simulink library "calcTetherEndNodesStates"  (R2018b)
settings: Solver=VariableStepAuto  StartTime=0.0  StopTime=10.0  RelTol=1e-3
undefined symbols (not defined in the file): attchPtMat, class_thr, numTethers
libraries: vrlib x1, eulAng2RotMat_ul x1
settings Model: Creator=Ayaz  LastModifiedBy=Ayaz

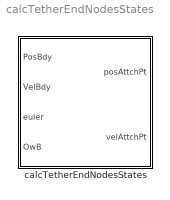
== system calcTetherEndNodesStates ==
  calcTetherEndNodesStates : Subsystem  TreatAsAtomicUnit=on  mask{thr_struct=class_thr, attach_point=Ground station}
      mask prompts: thr_struct "Tether class variable name"; attach_point "Choose attachment point"
      mask init:
      | sumTetherForcesAndMoments_init
      mask TypeOptions attach_point: Ground station | Lifting body

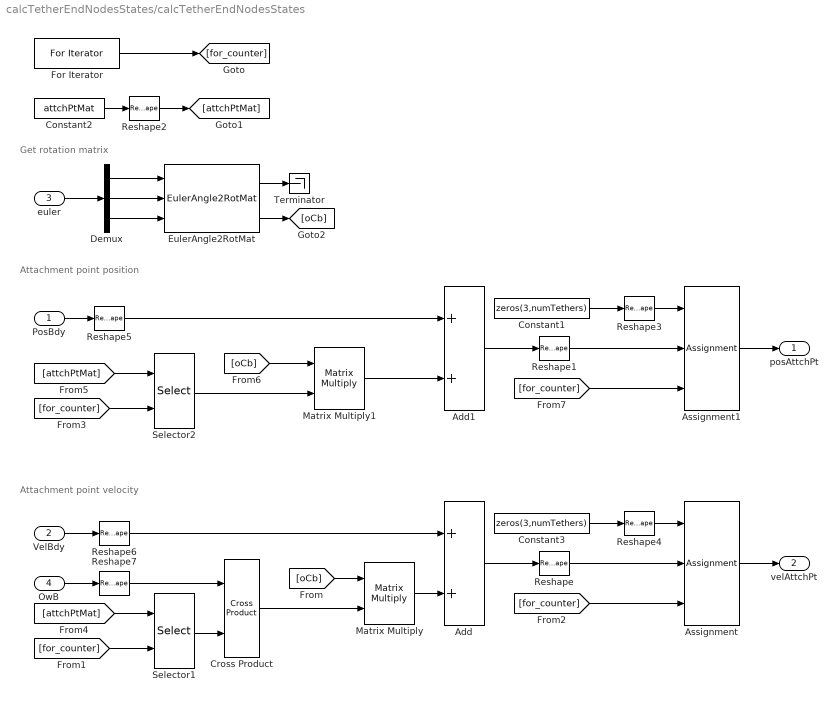
== system calcTetherEndNodesStates/calcTetherEndNodesStates ==
  note: Attachment point position
  note: Attachment point velocity
  note: Get rotation matrix
  PosBdy : Inport
  VelBdy : Inport  Port=2
  euler : Inport  Port=3
  OwB : Inport  Port=4
  Add : Sum
  Add1 : Sum
  Assignment : Assignment  NumberOfDimensions=2  DiagnosticForDimensions=Warning  IndexOptions=Assign all,Index vector (port)  Indices=1,1  OutputSizes=1,1
  Assignment1 : Assignment  NumberOfDimensions=2  DiagnosticForDimensions=Warning  IndexOptions=Assign all,Index vector (port)  Indices=1,1  OutputSizes=1,1
  Constant1 : Constant  Value=zeros(3,numTethers)  VectorParams1D=off
  Constant2 : Constant  Value=attchPtMat  VectorParams1D=off
  Constant3 : Constant  Value=zeros(3,numTethers)  VectorParams1D=off
  Cross Product : vrlib/Utilities/Cross Product
      settings: SourceProductBaseCode=VR
  Demux : Demux  Outputs=3
  EulerAngle2RotMat : eulAng2RotMat_ul/EulerAngle2RotMat  SystemSampleTime=-1
  For Iterator : ForIterator  IterationLimit=numTethers
  Matrix Multiply : Product  Multiplication=Matrix(*)
  Matrix Multiply1 : Product  Multiplication=Matrix(*)
  Reshape{,1,5..7} (5 alike) : Reshape  OutputDimensionality=Column vector (2-D)
  Reshape2 : Reshape  OutputDimensionality=Customize  OutputDimensions=[3,numTethers]
  Reshape3 : Reshape  OutputDimensionality=Customize  OutputDimensions=[3,numTethers]
  Reshape4 : Reshape  OutputDimensionality=Customize  OutputDimensions=[3,numTethers]
  Selector1 : Selector  NumberOfDimensions=2  InputPortWidth=3  IndexOptions=Select all,Index vector (port)  Indices=[1 3],1  OutputSizes=1,1
  Selector2 : Selector  NumberOfDimensions=2  InputPortWidth=3  IndexOptions=Select all,Index vector (port)  Indices=[1 3],1  OutputSizes=1,1
  Terminator : Terminator
  posAttchPt : Outport
  velAttchPt : Outport  Port=2
  wires:
  euler/1 -> Demux/1
  Demux/1 -> EulerAngle2RotMat/1
  Demux/2 -> EulerAngle2RotMat/2
  Demux/3 -> EulerAngle2RotMat/3
  EulerAngle2RotMat/1 -> Terminator/1
  EulerAngle2RotMat/2 -> [oCb]
  For Iterator/1 -> [for_counter]
  [for_counter] -> Selector1/2
  Selector1/1 -> Cross Product/2
  OwB/1 -> Reshape7/1
  [oCb] -> Matrix Multiply/1
  Cross Product/1 -> Matrix Multiply/2
  Matrix Multiply/1 -> Add/2
  VelBdy/1 -> Reshape6/1
  [for_counter] -> Assignment/3
  Reshape/1 -> Assignment/2
  Assignment/1 -> velAttchPt/1
  Add/1 -> Reshape/1
  Selector2/1 -> Matrix Multiply1/2
  [for_counter] -> Selector2/2
  [attchPtMat] -> Selector2/1
  [attchPtMat] -> Selector1/1
  [oCb] -> Matrix Multiply1/1
  Matrix Multiply1/1 -> Add1/2
  PosBdy/1 -> Reshape5/1
  Reshape1/1 -> Assignment1/2
  [for_counter] -> Assignment1/3
  Add1/1 -> Reshape1/1
  Assignment1/1 -> posAttchPt/1
  Constant2/1 -> Reshape2/1
  Reshape2/1 -> [attchPtMat]
  Constant1/1 -> Reshape3/1
  Reshape3/1 -> Assignment1/1
  Constant3/1 -> Reshape4/1
  Reshape4/1 -> Assignment/1
  Reshape5/1 -> Add1/1
  Reshape6/1 -> Add/1
  Reshape7/1 -> Cross Product/1
